simulink model "Target_Control_System"  (R2021b)
settings: Solver=FixedStepDiscrete  StartTime=0.0  StopTime=5  RelTol=1e-3
PreLoadFcn:
  | RTWConfigurationCB('preloadfcn', bdroot);
PostLoadFcn:
  | load('configuration/data_struct.mat');
  | load('configuration/fluxMaps_propMotor.mat');
  | load('configuration/parameterInit_PROP.mat');
  | load('configuration/parameterInit_PUMP.mat');
  | load('configuration/parameterInit_PITCH.mat');
  | load('configuration/parameterInit_TILT.mat');
  | %load('configuration/base_workspace_signal_definition.mat');
  | %load('resolvedatastores_to_baseworkspace_for_faster_simulation.mat');
model workspace (MAT data in the model file):
  SIMULATION_OPTIONS : Simulink.Parameter (value not decoded)
  TARGET_CODE_GEN : Simulink.Parameter (value not decoded)
  TCS_SAMPLE_FREQ_HZ : Simulink.Parameter (value not decoded)
symbols that are objects in the model workspace (value not decoded): TARGET_CODE_GEN, TCS_SAMPLE_FREQ_HZ
undefined symbols (not defined in the file): A_DQ_REF_LPF_INIT__PITCH, A_DQ_REF_LPF_INIT__PROP, A_DQ_REF_LPF_INIT__PUMP, A_DQ_REF_LPF_INIT__TILT, A_OBSERVER_CONFIDENCE_INIT__PITCH, A_OBSERVER_CONFIDENCE_INIT__PROP, A_OBSERVER_CONFIDENCE_INIT__PUMP, A_OBSERVER_CONFIDENCE_INIT__TILT, ACTUATOR_MAX_ANGLE_TRIP__PITCH, ACTUATOR_MIN_ANGLE_TRIP__PITCH, ACTUATOR_POS_SENSOR_INV_DIRECTION__PITCH, ACTUATOR_POS_SENSOR_INV_DIRECTION__TILT, ACTUATOR_POS_SENSOR_OFFSET__PITCH, ACTUATOR_POS_SENSOR_OFFSET__TILT, ADC_scaler1_baseaddr_TILT, ADC_SCALER_FLOAT_TO_FIXPOINT_EXPANSION, ANGLE_ELEC_FROM_SENSOR_OFFSET_INIT__PITCH, ANGLE_ELEC_FROM_SENSOR_OFFSET_INIT__PROP, ANGLE_ELEC_FROM_SENSOR_OFFSET_INIT__PUMP, ANGLE_ELEC_FROM_SENSOR_OFFSET_INIT__TILT, AUTO_CLEAR_FAULTS_ENABLED__PITCH, AUTO_CLEAR_FAULTS_ENABLED__PROP, AUTO_CLEAR_FAULTS_ENABLED__PUMP, AUTO_CLEAR_FAULTS_ENABLED__TILT, AUTO_CLEAR_FAULTS_WAIT_TICKS__PITCH, AUTO_CLEAR_FAULTS_WAIT_TICKS__PROP, AUTO_CLEAR_FAULTS_WAIT_TICKS__PUMP, AUTO_CLEAR_FAULTS_WAIT_TICKS__TILT, AUTO_I_ZERO_IDLE_TICKS__PITCH, AUTO_I_ZERO_IDLE_TICKS__PROP, AUTO_I_ZERO_IDLE_TICKS__PUMP, AUTO_I_ZERO_IDLE_TICKS__TILT, AUTO_I_ZERO_OFFSET_IDC_THRESHOLD__PITCH, AUTO_I_ZERO_OFFSET_IDC_THRESHOLD__PROP, AUTO_I_ZERO_OFFSET_IDC_THRESHOLD__PUMP, AUTO_I_ZERO_OFFSET_IDC_THRESHOLD__TILT, AUTO_I_ZERO_OFFSET_IPH_THRESHOLD__PITCH, AUTO_I_ZERO_OFFSET_IPH_THRESHOLD__PROP, AUTO_I_ZERO_OFFSET_IPH_THRESHOLD__PUMP, AUTO_I_ZERO_OFFSET_IPH_THRESHOLD__TILT, AUTO_SENSORLESS_SWITCHOVER_DISABLE_OMEGA, AUTO_SENSORLESS_SWITCHOVER_ENABLE_OMEGA, AUTO_SENSORLESS_SWITCHOVER_MIN_CONFIDENCE, AUXILIARY_PROTECTION_UNIT_BASEADDR__TILT, blanking_max_error_omega_INIT_PITCH, blanking_max_error_omega_INIT_TILT, blanking_max_error_position_INIT_PITCH, blanking_max_error_position_INIT_TILT, BRUTE_START_I_Q_REF_RAMP_SPEED__PITCH, BRUTE_START_I_Q_REF_RAMP_SPEED__PROP, BRUTE_START_I_Q_REF_RAMP_SPEED__PUMP, BRUTE_START_I_Q_REF_RAMP_SPEED__TILT, CONTROL_LOOP_DT_INIT__PITCH, CONTROL_LOOP_DT_INIT__PROP, CONTROL_LOOP_DT_INIT__PUMP, CONTROL_LOOP_DT_INIT__TILT, CORRECTION_FILTER_SCALE__PITCH, CORRECTION_FILTER_SCALE__PROP, CORRECTION_FILTER_SCALE__PUMP, CORRECTION_FILTER_SCALE__TILT ... (+458)
libraries: simulink x178, Reusables_Lib x24
(part 37 of 47)

== system Target_Control_System/Target_Control_System/MainLoop/pitchMotor_mainLoop/mainTask_pitch/motorTaskMainFastStep()/Control Loops - Pitch/Speed Controller Pitch/Enabled Subsystem1 ==
  oRampDataOmegaERef_.fRampOut : Inport
  Enable : EnablePort
  Constant2 : Constant  OutDataTypeStr=single  SampleTime=-1
  Data Store Read1 : DataStoreRead  DataStoreName=oPitch  DataStoreElements=oPitch.oMot_.oParam_.oPiDataRpm_.oParameter_.fKp_  IndexOptions=Index vector (dialog)  Indices=1  OutputSizes=1
  Data Store Read11 : DataStoreRead  DataStoreName=oPitch  DataStoreElements=oPitch.oMot_.oParam_.oPiDataRpm_.oParameter_.fIntMax_  IndexOptions=Index vector (dialog)  Indices=1  OutputSizes=1
  Data Store Read13 : DataStoreRead  DataStoreName=oPitch  DataStoreElements=oPitch.oMot_.oParam_.oPiDataRpm_.oParameter_.fOutMin_  IndexOptions=Index vector (dialog)  Indices=1  OutputSizes=1
  Data Store Read2 : DataStoreRead  DataStoreName=oPitch  DataStoreElements=oPitch.oMot_.oParam_.oPiDataRpm_.oParameter_.fKi_  IndexOptions=Index vector (dialog)  Indices=1  OutputSizes=1
  Data Store Read25 : DataStoreRead  DataStoreName=oPitch  DataStoreElements=oPitch.oMot_.oParam_.oPiDataRpm_.oParameter_.fOutMax_  IndexOptions=Index vector (dialog)  Indices=1  OutputSizes=1
  Data Store Read26 : DataStoreRead  DataStoreName=oPitch  DataStoreElements=oPitch.oMot_.oParam_.oPiDataRpm_.fState_  IndexOptions=Index vector (dialog)  Indices=1  OutputSizes=1
  Data Store Read27 : DataStoreRead  DataStoreName=oPitch  DataStoreElements=oPitch.oMot_.oIn_.fOmegaEObserverLpf2_  IndexOptions=Index vector (dialog)  Indices=1  OutputSizes=1
  Data Store Read5 : DataStoreRead  DataStoreName=oPitch  DataStoreElements=oPitch.oMot_.oParam_.oPiDataRpm_.oParameter_.fLoopDt_  IndexOptions=Index vector (dialog)  Indices=1  OutputSizes=1
  Data Store Read6 : DataStoreRead  DataStoreName=oPitch  DataStoreElements=oPitch.oMot_.oParam_.oPiDataRpm_.oParameter_.fIntMin_  IndexOptions=Index vector (dialog)  Indices=1  OutputSizes=1
  Data Store Write4 : DataStoreWrite  DataStoreName=oPitch  DataStoreElements=oPitch.oMot_.oState_.fIqRefFromSpeedController_  IndexOptions=Index vector (dialog)  Indices=1  OutputSizes=1
  Data Store Write6 : DataStoreWrite  DataStoreName=oPitch  DataStoreElements=oPitch.oMot_.oParam_.oPiDataRpm_.fState_  IndexOptions=Index vector (dialog)  Indices=1  OutputSizes=1
  PI Iq Current Controller : Subsystem
  fIqRefFromSpeedController : Outport
  wires:
  PI Iq Current Controller/1(fOutput) -> Data Store Write4/1, fIqRefFromSpeedController/1
  PI Iq Current Controller/2(*fpState) -> Data Store Write6/1
  oRampDataOmegaERef_.fRampOut/1 -> PI Iq Current Controller/1(fTarget)
  Data Store Read27/1 -> PI Iq Current Controller/2(fActual)
  Constant2/1 -> PI Iq Current Controller/5(fScale)
  Data Store Read25/1 -> PI Iq Current Controller/8(fOutMax)
  Data Store Read13/1 -> PI Iq Current Controller/10(fOutMin)
  Data Store Read11/1 -> PI Iq Current Controller/7(fIntMax)
  Data Store Read6/1 -> PI Iq Current Controller/9(fIntMin)
  Data Store Read5/1 -> PI Iq Current Controller/6(fLoopDt)
  Data Store Read2/1 -> PI Iq Current Controller/4(fKi)
  Data Store Read1/1 -> PI Iq Current Controller/3(fKp)

== system Target_Control_System/Target_Control_System/MainLoop/pitchMotor_mainLoop/mainTask_pitch/motorTaskMainFastStep()/Control Loops - Pitch/Speed Controller Pitch/Set Iq Ref Pitch ==
  note: // Run a low pass filter on the reference output from the speed controller.
      | // Main motivation: this is for the other inverter in dual motor servo loops, where the other inverter runs in torque
      | // mirror mode. The comms bandwidth to the other inverter is slower than the control loop. Without filter, aliasing will
      | // happen. (Example: on a quick motor deceleration there might be a brief high torque spike. If exactly this spike gets
      | // communicated across, the other inverter will apply this torque for much longer, essentially causing the inverters to
      | // fight for a few cycles.)
  fIqRefFromSpeedController : Inport
  Enable : EnablePort
  Data Store Read : DataStoreRead  DataStoreName=oPitch  DataStoreElements=oPitch.oMot_.oState_.oFilterDataForSpeedControlIqRef_.afConstantsA_.h0  IndexOptions=Index vector (dialog)  Indices=1  OutputSizes=1
  Data Store Read1 : DataStoreRead  DataStoreName=oPitch  DataStoreElements=oPitch.oMot_.oState_.oFilterDataForSpeedControlIqRef_.afConstantsA_.h1  IndexOptions=Index vector (dialog)  Indices=1  OutputSizes=1
  Data Store Read2 : DataStoreRead  DataStoreName=oPitch  DataStoreElements=oPitch.oMot_.oState_.oFilterDataForSpeedControlIqRef_.afConstantsA_.h2  IndexOptions=Index vector (dialog)  Indices=1  OutputSizes=1
  Data Store Read3 : DataStoreRead  DataStoreName=oPitch  DataStoreElements=oPitch.oMot_.oState_.oFilterDataForSpeedControlIqRef_.afConstantsB_.h0  IndexOptions=Index vector (dialog)  Indices=1  OutputSizes=1
  Data Store Read4 : DataStoreRead  DataStoreName=oPitch  DataStoreElements=oPitch.oMot_.oState_.oFilterDataForSpeedControlIqRef_.afConstantsB_.h1  IndexOptions=Index vector (dialog)  Indices=1  OutputSizes=1
  Data Store Read5 : DataStoreRead  DataStoreName=oPitch  DataStoreElements=oPitch.oMot_.oState_.oFilterDataForSpeedControlIqRef_.afConstantsB_.h2  IndexOptions=Index vector (dialog)  Indices=1  OutputSizes=1
  Data Store Read6 : DataStoreRead  DataStoreName=oPitch  DataStoreElements=oPitch.oMot_.oState_.oFilterDataForSpeedControlIqRef_.afPreviousInputs_.h0  IndexOptions=Index vector (dialog)  Indices=1  OutputSizes=1
  Data Store Read7 : DataStoreRead  DataStoreName=oPitch  DataStoreElements=oPitch.oMot_.oState_.oFilterDataForSpeedControlIqRef_.afPreviousInputs_.h1  IndexOptions=Index vector (dialog)  Indices=1  OutputSizes=1
  Data Store Read8 : DataStoreRead  DataStoreName=oPitch  DataStoreElements=oPitch.oMot_.oState_.oFilterDataForSpeedControlIqRef_.afPreviousOutputs_.h0  IndexOptions=Index vector (dialog)  Indices=1  OutputSizes=1
  Data Store Read9 : DataStoreRead  DataStoreName=oPitch  DataStoreElements=oPitch.oMot_.oState_.oFilterDataForSpeedControlIqRef_.afPreviousOutputs_.h1  IndexOptions=Index vector (dialog)  Indices=1  OutputSizes=1
  Data Store Write1 : DataStoreWrite  DataStoreName=oPitch  DataStoreElements=oPitch.oMot_.oState_.oFilterDataForSpeedControlIqRef_.fFilterOutput_  IndexOptions=Index vector (dialog)  Indices=1  OutputSizes=1
  Data Store Write2 : DataStoreWrite  DataStoreName=oPitch  DataStoreElements=oPitch.oMot_.oState_.oFilterDataForSpeedControlIqRef_.afPreviousOutputs_.h0  IndexOptions=Index vector (dialog)  Indices=1  OutputSizes=1
  Data Store Write3 : DataStoreWrite  DataStoreName=oPitch  DataStoreElements=oPitch.oMot_.oState_.oFilterDataForSpeedControlIqRef_.afPreviousOutputs_.h1  IndexOptions=Index vector (dialog)  Indices=1  OutputSizes=1
  Data Store Write4 : DataStoreWrite  DataStoreName=oPitch  DataStoreElements=oPitch.oMot_.oState_.oFilterDataForSpeedControlIqRef_.afPreviousInputs_.h0  IndexOptions=Index vector (dialog)  Indices=1  OutputSizes=1
  Data Store Write5 : DataStoreWrite  DataStoreName=oPitch  DataStoreElements=oPitch.oMot_.oState_.oFilterDataForSpeedControlIqRef_.afPreviousInputs_.h1  IndexOptions=Index vector (dialog)  Indices=1  OutputSizes=1
  Data Store Write6 : DataStoreWrite  DataStoreName=oPitch  DataStoreElements=oPitch.oMot_.oState_.fIqRefBeforeRamp_  IndexOptions=Index vector (dialog)  Indices=1  OutputSizes=1
  softwareIirFilterStep() : Subsystem
  wires:
  fIqRefFromSpeedController/1 -> softwareIirFilterStep()/1(newInput), Data Store Write6/1
  softwareIirFilterStep()/1(*afPreviousInputs1) -> Data Store Write5/1
  softwareIirFilterStep()/2(*afPreviousInputs0) -> Data Store Write4/1
  softwareIirFilterStep()/3(*afPreviousOutputs1) -> Data Store Write3/1
  softwareIirFilterStep()/4(*afPreviousOutputs0) -> Data Store Write2/1
  softwareIirFilterStep()/5(fFilterOutput) -> Data Store Write1/1
  Data Store Read6/1 -> softwareIirFilterStep()/8(afPreviousInputs0)
  Data Store Read7/1 -> softwareIirFilterStep()/9(afPreviousInputs1)
  Data Store Read8/1 -> softwareIirFilterStep()/10(afPreviousOutputs0)
  Data Store Read9/1 -> softwareIirFilterStep()/11(afPreviousOutputs1)
  Data Store Read2/1 -> softwareIirFilterStep()/7(afConstantsA2)
  Data Store Read1/1 -> softwareIirFilterStep()/6(afConstantsA1)
  Data Store Read/1 -> softwareIirFilterStep()/5(afConstantsA0)
  Data Store Read3/1 -> softwareIirFilterStep()/2(afConstantsB0)
  Data Store Read4/1 -> softwareIirFilterStep()/3(afConstantsB1)
  Data Store Read5/1 -> softwareIirFilterStep()/4(afConstantsB2)

== system Target_Control_System/Target_Control_System/MainLoop/pitchMotor_mainLoop/mainTask_pitch/motorTaskMainFastStep()/Mechanical System - Pitch/processSensors(&oPitch)/Auxiliary sensor ==
  note: // Only process this if the sensor is actually there (mostly to save time for the QI).
  Enable : EnablePort
  Add2 : Sum
  Add4 : Sum
  Constant16 : Constant  Value=pi  OutDataTypeStr=single  SampleTime=-1
  Constant17 : Constant  Value=2*pi  OutDataTypeStr=single  SampleTime=-1
  Constant3 : Constant  Value=pi  OutDataTypeStr=single  SampleTime=-1
  Constant6 : Constant  Value=2*pi  OutDataTypeStr=single  SampleTime=-1
  Data Store Read67 : DataStoreRead  DataStoreName=oPitch  DataStoreElements=oPitch.oMot_.oState_.oPosSensor_.iAuxiliarySensorInverseDirection_  IndexOptions=Index vector (dialog)  Indices=1  OutputSizes=1
  Data Store Read68 : DataStoreRead  DataStoreName=oPitch  DataStoreElements=oPitch.oMot_.oIn_.oAdcData_.fAuxiliaryEncoderFloat_  IndexOptions=Index vector (dialog)  Indices=1  OutputSizes=1
  Data Store Read91 : DataStoreRead  DataStoreName=oPitch  DataStoreElements=oPitch.oMot_.oState_.oPosSensor_.fAuxiliarySensorOffsetAngle_  IndexOptions=Index vector (dialog)  Indices=1  OutputSizes=1
  Data Store Write37 : DataStoreWrite  DataStoreName=oPitch  DataStoreElements=oPitch.oMot_.oState_.oPosSensor_.fAuxiliaryAngleFromSensor_  IndexOptions=Index vector (dialog)  Indices=1  OutputSizes=1
  Subtract3 : Sum  Inputs=+-
  Subtract4 : Sum  Inputs=+-
  Subtract5 : Sum  Inputs=-+
  Switch10 : Switch  Threshold=-pi/2.0
  Switch8 : Switch  Criteria=u2 > Threshold
  Switch9 : Switch  Criteria=u2 > Threshold  Threshold=1.5*pi
  wires:
  Switch9/1 -> Data Store Write37/1
  Data Store Read91/1 -> Add2/1
  Constant16/1 -> Subtract4/2
  Add4/1 -> Switch10/3
  Add2/1 -> Subtract5/2, Add4/1, Switch10/2, Switch10/1, Switch9/2
  Data Store Read68/1 -> Subtract3/2, Subtract4/1
  Subtract4/1 -> Switch8/3
  Data Store Read67/1 -> Switch8/2
  Subtract5/1 -> Switch9/1
  Constant6/1 -> Add4/2
  Switch10/1 -> Switch9/3
  Subtract3/1 -> Switch8/1
  Constant17/1 -> Subtract5/1
  Switch8/1 -> Add2/2
  Constant3/1 -> Subtract3/1

== system Target_Control_System/Target_Control_System/MainLoop/pitchMotor_mainLoop/mainTask_pitch/motorTaskMainFastStep()/Mechanical System - Pitch/processSensors(&oPitch)/Input (motor) side sensor ==
  note: // Ensure the angle is within -pi/2 to pi*1.5 (no loop needed, assuming 'fActuatorSensorOffsetAngle_' is within -pi to pi)
      |    // The reason for this 'skewed' wrap around angle: the tilt sensor on the linkage style tilts moves between 0 and 200 deg,
      |    // so it'd be mighty convenient if it doesn't wrap around at 180 deg. The flaps have a similar situation.
      |    // For pivot style tilt and VP, the sensor moves between -15 deg and 100 deg at most, so the the shifted wrapping point is a non-issue.
  note: // In the tilt motor on nacelles 1 and 4-6, the sensor read head is mounted to the gearbox output shaft.
      | // For every full motor rotation, the read head moves by 1/160*360 degrees = 2.25 degrees w.r.t the stator.
      | // (So with our 20 pole pairs, that is 45 degrees electrical.)
      | // We have to adjust the offset for this.
  note: //Note to future self: there is a slim chance that 'opStates->oPosSensor_.oGbx_.fCurrentOutputAngle_'
      | may need to be multiplied by -1.0F for certain hardware assemblies. Just keep it in mind.
  " " : Subsystem
  Add5 : Sum
  Add6 : Sum
  Compute Speed From Sensor : Subsystem
  Constant15 : Constant  Value=pi  OutDataTypeStr=single  SampleTime=-1
  Constant18 : Constant  Value=pi  OutDataTypeStr=single  SampleTime=-1
  Data Store Read101 : DataStoreRead  DataStoreName=oPitch  DataStoreElements=oPitch.oMot_.oState_.oPosSensor_.iMotorSensorInverseDirection_  IndexOptions=Index vector (dialog)  Indices=1  OutputSizes=1
  Data Store Read102 : DataStoreRead  DataStoreName=oPitch  DataStoreElements=oPitch.oMot_.oIn_.oAdcData_.fMotorEncoderFloat_  IndexOptions=Index vector (dialog)  Indices=1  OutputSizes=1
  Data Store Read70 : DataStoreRead  DataStoreName=oPitch  DataStoreElements=oPitch.oMot_.oState_.oPosSensor_.fAngleElecFromSensorOffset_  IndexOptions=Index vector (dialog)  Indices=1  OutputSizes=1
  Data Store Read72 : DataStoreRead  DataStoreName=oPitch  DataStoreElements=oPitch.oMot_.oParam_.fOneOverSensorPolepairs_  IndexOptions=Index vector (dialog)  Indices=1  OutputSizes=1
  Data Store Read85 : DataStoreRead  DataStoreName=oPitch  DataStoreElements=oPitch.oMot_.oState_.oPosSensor_.iAngleElecFromSensorNumOfIdenticalValues_  IndexOptions=Index vector (dialog)  Indices=1  OutputSizes=1
  Data Store Read96 : DataStoreRead  DataStoreName=oPitch  DataStoreElements=oPitch.oMot_.oState_.oPosSensor_.iTiltReadheadCompensationEnabled_  IndexOptions=Index vector (dialog)  Indices=1  OutputSizes=1
  Data Store Read98 : DataStoreRead  DataStoreName=oPitch  DataStoreElements=oPitch.oMot_.oParam_.fPolePairs_  IndexOptions=Index vector (dialog)  Indices=1  OutputSizes=1
  Data Store Write1 : DataStoreWrite  DataStoreName=oPitch  DataStoreElements=oPitch.oMot_.oState_.oPosSensor_.fAngleElecFromSensor_  IndexOptions=Index vector (dialog)  Indices=1  OutputSizes=1
  Data Store Write38 : DataStoreWrite  DataStoreName=oPitch  DataStoreElements=oPitch.oMot_.oState_.oPosSensor_.fAngleMechMotorFromSensor_  IndexOptions=Index vector (dialog)  Indices=1  OutputSizes=1
  Data Store Write40 : DataStoreWrite  DataStoreName=oPitch  DataStoreElements=oPitch.oMot_.oState_.oPosSensor_.fOmegaEFromSensor_  IndexOptions=Index vector (dialog)  Indices=1  OutputSizes=1
  Data Store Write41 : DataStoreWrite  DataStoreName=oPitch  DataStoreElements=oPitch.oMot_.oState_.oPosSensor_.fAngleElecFromSensorPrevious_  IndexOptions=Index vector (dialog)  Indices=1  OutputSizes=1
  Data Store Write42 : DataStoreWrite  DataStoreName=oPitch  DataStoreElements=oPitch.oMot_.oState_.oPosSensor_.iAngleMechToElecWrappings_  IndexOptions=Index vector (dialog)  Indices=1  OutputSizes=1
  Product : Product  Inputs=3
  Stuck Sensor Detection : Subsystem
  Subtract6 : Sum  Inputs=+-
  Subtract7 : Sum  Inputs=+-
  Switch14 : Switch  Criteria=u2 > Threshold
  Switch16 : Switch  Criteria=u2 > Threshold
  Unit Delay : UnitDelay  SampleTime=-1  HasFrameUpgradeWarning=on
  updateGbxOutput : Subsystem
  wires:
  Switch16/1 -> Product/1
  Data Store Read96/1 -> Switch16/2
  Data Store Read70/1 -> Add6/2
  Data Store Read101/1 -> Switch14/2
  Add6/1 -> " "/1(input_angle)  "angle_elec_unwrapped"
  Add5/1 -> Switch16/1
  Switch14/1 -> Data Store Write38/1, updateGbxOutput/1(fNewInputAngle), Switch16/3, Add5/2  "fAngleMechMotorFromSensor"
  " "/2(wrapped_angle) -> Unit Delay/1, Compute Speed From Sensor/2(fAngleElecFromSensor), Stuck Sensor Detection/1(fAngleElecFromSensor), Data Store Write1/1  "fAngleElecFromSensor"
  " "/1(rev_count) -> Data Store Write42/1
  Data Store Read102/1 -> Subtract7/1, Subtract6/2  "fMotorEncoderFloat"
  Data Store Read72/1 -> Product/3
  Product/1 -> Add6/1
  Data Store Read85/1 -> Stuck Sensor Detection/2(NumOfIdenticalValues)
  Compute Speed From Sensor/1(fOmegaEFromSensor) -> Data Store Write40/1
  Constant15/1 -> Subtract7/2
  Subtract6/1 -> Switch14/1
  Data Store Read98/1 -> Product/2
  Unit Delay/1 -> Stuck Sensor Detection/3(fAngleElecFromSensorPrevious), Compute Speed From Sensor/1(fAngleElecFromSensorPrevious)
  Compute Speed From Sensor/2(AngleCurrent) -> Data Store Write41/1
  Constant18/1 -> Subtract6/1
  updateGbxOutput/1(fCurrentOutputAngle) -> Add5/1
  Subtract7/1 -> Switch14/3

== system Target_Control_System/Target_Control_System/MainLoop/pitchMotor_mainLoop/mainTask_pitch/motorTaskMainFastStep()/Mechanical System - Pitch/processSensors(&oPitch)/Output (actuator) side sensor ==
  note: // Ensure the angle is within -pi/2 to pi*1.5 (no loop needed, assuming 'fActuatorSensorOffsetAngle_' is within -pi to pi)
      |    // The reason for this 'skewed' wrap around angle: the tilt sensor on the linkage style tilts moves between 0 and 200 deg,
      |    // so it'd be mighty convenient if it doesn't wrap around at 180 deg. The flaps have a similar situation.
      |    // For pivot style tilt and VP, the sensor moves between -15 deg and 100 deg at most, so the the shifted wrapping point is a non-issue.
  Add : Sum
  Add4 : Sum
  Constant16 : Constant  Value=pi  OutDataTypeStr=single  SampleTime=-1
  Constant17 : Constant  Value=2*pi  OutDataTypeStr=single  SampleTime=-1
  Constant3 : Constant  Value=pi  OutDataTypeStr=single  SampleTime=-1
  Constant6 : Constant  Value=2*pi  OutDataTypeStr=single  SampleTime=-1
  Data Store Read67 : DataStoreRead  DataStoreName=oPitch  DataStoreElements=oPitch.oMot_.oState_.oPosSensor_.iActuatorSensorInverseDirection_  IndexOptions=Index vector (dialog)  Indices=1  OutputSizes=1
  Data Store Read68 : DataStoreRead  DataStoreName=oPitch  DataStoreElements=oPitch.oMot_.oIn_.oAdcData_.fOutputEncoderFloat_  IndexOptions=Index vector (dialog)  Indices=1  OutputSizes=1
  Data Store Read91 : DataStoreRead  DataStoreName=oPitch  DataStoreElements=oPitch.oMot_.oState_.oPosSensor_.fActuatorSensorOffsetAngle_  IndexOptions=Index vector (dialog)  Indices=1  OutputSizes=1
  Data Store Write37 : DataStoreWrite  DataStoreName=oPitch  DataStoreElements=oPitch.oMot_.oState_.oPosSensor_.fActuatorAngleFromSensor_  IndexOptions=Index vector (dialog)  Indices=1  OutputSizes=1
  Subtract : Sum  Inputs=+-
  Subtract1 : Sum  Inputs=+-
  Subtract2 : Sum  Inputs=-+
  Switch10 : Switch  Threshold=-pi/2.0
  Switch8 : Switch  Criteria=u2 > Threshold
  Switch9 : Switch  Criteria=u2 > Threshold  Threshold=1.5*pi
  wires:
  Constant6/1 -> Add4/2
  Constant17/1 -> Subtract2/1
  Subtract2/1 -> Switch9/1
  Data Store Read91/1 -> Add/1
  Subtract/1 -> Switch8/1
  Switch10/1 -> Switch9/3
  Switch9/1 -> Data Store Write37/1
  Constant3/1 -> Subtract/1
  Constant16/1 -> Subtract1/2
  Data Store Read68/1 -> Subtract/2, Subtract1/1
  Subtract1/1 -> Switch8/3
  Data Store Read67/1 -> Switch8/2
  Switch8/1 -> Add/2
  Add/1 -> Subtract2/2, Add4/1, Switch10/2, Switch10/1, Switch9/2
  Add4/1 -> Switch10/3

== system Target_Control_System/Target_Control_System/MainLoop/pitchMotor_mainLoop/mainTask_pitch/motorTaskMainFastStep()/Motor Acceleration - Pitch/First filter stage/softwareIirFilterStep() ==
  newInput : Inport
  afConstantsB0 : Inport  Port=2
  afConstantsB1 : Inport  Port=3
  afConstantsB2 : Inport  Port=4
  afConstantsA0 : Inport  Port=5
  afConstantsA1 : Inport  Port=6
  afConstantsA2 : Inport  Port=7
  afPreviousInputs0 : Inport  Port=8
  afPreviousInputs1 : Inport  Port=9
  afPreviousOutputs0 : Inport  Port=10
  afPreviousOutputs1 : Inport  Port=11
  Add : Sum  Inputs=+++--
  Constant : Constant  Value=0  OutDataTypeStr=single  SampleTime=-1
  Constant1 : Constant  Value=0  OutDataTypeStr=single  SampleTime=-1
  Divide{,1..5} (6 alike) : Product  Inputs=**
  IsInf : RelationalOperator  Operator=isInf  OutDataTypeStr=boolean  RndMeth=Simplest
  IsInf1 : RelationalOperator  Operator=isInf  OutDataTypeStr=boolean  RndMeth=Simplest
  IsNaN : RelationalOperator  Operator=isNaN  OutDataTypeStr=boolean  RndMeth=Simplest
  IsNaN1 : RelationalOperator  Operator=isNaN  OutDataTypeStr=boolean  RndMeth=Simplest
  Switch{,1..3} (4 alike) : Switch  Criteria=u2 > Threshold
  *afPreviousInputs1 : Outport
  *afPreviousInputs0 : Outport  Port=2
  *afPreviousOutputs1 : Outport  Port=3
  *afPreviousOutputs0 : Outport  Port=4
  fFilterOutput : Outport  Port=5
  wires:
  Switch3/1 -> Divide5/1, *afPreviousOutputs0/1
  IsInf1/1 -> Switch3/2
  IsNaN1/1 -> Switch2/2
  Constant1/1 -> Switch2/1, Switch3/1
  Switch2/1 -> IsInf1/1, Switch3/3
  Add/1 -> IsNaN1/1, Switch2/3  "fOutput"
  Switch1/1 -> Divide/1, *afPreviousInputs0/1
  Switch/1 -> IsInf/1, Switch1/3
  IsInf/1 -> Switch1/2
  Constant/1 -> Switch/1, Switch1/1
  IsNaN/1 -> Switch/2
  Divide5/1 -> fFilterOutput/1
  afConstantsA0/1 -> Divide5/2
  afPreviousOutputs1/1 -> Divide4/1
  afConstantsA2/1 -> Divide4/2
  afPreviousOutputs0/1 -> Divide3/1, *afPreviousOutputs1/1
  afConstantsA1/1 -> Divide3/2
  afPreviousInputs1/1 -> Divide2/1
  afConstantsB2/1 -> Divide2/2
  Divide4/1 -> Add/5
  Divide3/1 -> Add/4
  Divide/1 -> Add/1
  Divide1/1 -> Add/2
  Divide2/1 -> Add/3
  afPreviousInputs0/1 -> Divide1/1, *afPreviousInputs1/1
  afConstantsB1/1 -> Divide1/2
  newInput/1 -> IsNaN/1, Switch/3
  afConstantsB0/1 -> Divide/2

== system Target_Control_System/Target_Control_System/MainLoop/pitchMotor_mainLoop/mainTask_pitch/motorTaskMainFastStep()/Observer Confidence - Pitch/Automatic switching to sensorless/Switch to sensored?  ==
  fObserverConfidence : Inport
  Action Port : ActionPort
  Abs1 : Abs
  Data Store Read28 : DataStoreRead  DataStoreName=oPitch  DataStoreElements=oPitch.oMot_.oIn_.fOmegaEObserverRaw2_  IndexOptions=Index vector (dialog)  Indices=1  OutputSizes=1
  Data Store Read29 : DataStoreRead  DataStoreName=oPitch  DataStoreElements=oPitch.oMot_.oParam_.fAutoSensorlessSwitchoverDisableOmega_  IndexOptions=Index vector (dialog)  Indices=1  OutputSizes=1
  Data Store Read42 : DataStoreRead  DataStoreName=oPitch  DataStoreElements=oPitch.oMot_.oParam_.fAutoSensorlessSwitchoverMinConfidence_  IndexOptions=Index vector (dialog)  Indices=1  OutputSizes=1
  Less Than : RelationalOperator  Operator=<  OutDataTypeStr=boolean  RndMeth=Simplest
  Less Than1 : RelationalOperator  Operator=<  OutDataTypeStr=boolean  RndMeth=Simplest
  OR : Logic  Operator=OR  AllPortsSameDT=off  OutDataTypeStr=boolean
  Switch to sensored : Subsystem  TreatAsAtomicUnit=on
  wires:
  OR/1 -> Switch to sensored/Enable
  fObserverConfidence/1 -> Less Than1/1
  Data Store Read29/1 -> Less Than/2
  Data Store Read42/1 -> Less Than1/2
  Abs1/1 -> Less Than/1
  Less Than/1 -> OR/1
  Data Store Read28/1 -> Abs1/1
  Less Than1/1 -> OR/2

== system Target_Control_System/Target_Control_System/MainLoop/pitchMotor_mainLoop/mainTask_pitch/motorTaskMainFastStep()/Observer Confidence - Pitch/Automatic switching to sensorless/Switch to sensorless? ==
  fObserverConfidence : Inport
  Action Port : ActionPort
  Abs1 : Abs
  Data Store Read28 : DataStoreRead  DataStoreName=oPitch  DataStoreElements=oPitch.oMot_.oIn_.fOmegaEObserverRaw2_  IndexOptions=Index vector (dialog)  Indices=1  OutputSizes=1
  Data Store Read29 : DataStoreRead  DataStoreName=oPitch  DataStoreElements=oPitch.oMot_.oParam_.fAutoSensorlessSwitchoverEnableOmega_  IndexOptions=Index vector (dialog)  Indices=1  OutputSizes=1
  Data Store Read42 : DataStoreRead  DataStoreName=oPitch  DataStoreElements=oPitch.oMot_.oParam_.fAutoSensorlessSwitchoverMinConfidence_  IndexOptions=Index vector (dialog)  Indices=1  OutputSizes=1
  Less Than : RelationalOperator  Operator=>  OutDataTypeStr=boolean  RndMeth=Simplest
  Less Than1 : RelationalOperator  Operator=>  OutDataTypeStr=boolean  RndMeth=Simplest
  OR : Logic  AllPortsSameDT=off  OutDataTypeStr=boolean
  Switch to sensorless : Subsystem  TreatAsAtomicUnit=on
  wires:
  Less Than/1 -> OR/1
  Data Store Read42/1 -> Less Than1/2
  Less Than1/1 -> OR/2
  fObserverConfidence/1 -> Less Than1/1
  Data Store Read29/1 -> Less Than/2
  Data Store Read28/1 -> Abs1/1
  Abs1/1 -> Less Than/1
  OR/1 -> Switch to sensorless/Enable

== system Target_Control_System/Target_Control_System/MainLoop/pitchMotor_mainLoop/mainTask_pitch/motorTaskMainFastStep()/Software Overcurrent Protection - Pitch/checkForHwOvercurrents(&oPitch)/gateDriverStatus ==
  note: 1) Add Subsystem or Model blocks as valid variant choices.
      | 2) You cannot connect blocks at this level. At simulation, connectivity is automatically
      | determined, based on the active variant and port name matching.
  DoNotIncludeCustomCode : Subsystem  TreatAsAtomicUnit=on  VariantControl=TARGET_CODE_GEN == 0
  IncludeCustomCode : Subsystem  TreatAsAtomicUnit=on  VariantControl=(default)

== system Target_Control_System/Target_Control_System/MainLoop/propMotor_mainLoop/Decimation gate for 5000 Hz Prop/motorTaskProcessExternalSetpoints(&oProp)/Subsystem3/Subsystem/Subsystem ==
  Enable : EnablePort
  Data Store Read1 : DataStoreRead  DataStoreName=oProp  DataStoreElements=oProp.oMot_.oParam_.fIqSetpointMax_  IndexOptions=Index vector (dialog)  Indices=1  OutputSizes=1
  Data Store Read68 : DataStoreRead  DataStoreName=oProp  DataStoreElements=oProp.oMot_.oIn_.fIqSetpoint_  IndexOptions=Index vector (dialog)  Indices=1  OutputSizes=1
  Data Store Read74 : DataStoreRead  DataStoreName=oProp  DataStoreElements=oProp.oMot_.oParam_.fIqSetpointMax_  IndexOptions=Index vector (dialog)  Indices=1  OutputSizes=1
  Data Store Read81 : DataStoreRead  DataStoreName=oProp  DataStoreElements=oProp.oMot_.oParam_.fDynILimIntegratorLeakageFactor_  IndexOptions=Index vector (dialog)  Indices=1  OutputSizes=1
  Data Store Write19 : DataStoreWrite  DataStoreName=oProp  DataStoreElements=oProp.oMot_.oState_.fIqRefBeforeRamp_  IndexOptions=Index vector (dialog)  Indices=1  OutputSizes=1
  Dynamic Current Limiting Prop : Subsystem  TreatAsAtomicUnit=on
  Gain2 : Gain  Gain=-1
  Saturation Dynamic : simulink/Discontinuities/Saturation Dynamic  OutMin=[]  OutMax=[]  OutDataTypeStr=Inherit: Same as second input  OutDataType=fixdt(1, 16)  OutScaling=2^-10  DoSatur=off
  Switch4 : Switch  Criteria=u2 > Threshold
  wires:
  Dynamic Current Limiting Prop/1(fIqRefBeforeRamp_) -> Switch4/1
  Switch4/1 -> Data Store Write19/1
  Data Store Read81/1 -> Dynamic Current Limiting Prop/Enable, Switch4/2
  Gain2/1 -> Saturation Dynamic/3
  Data Store Read74/1 -> Saturation Dynamic/1
  Data Store Read68/1 -> Saturation Dynamic/2
  Data Store Read1/1 -> Gain2/1
  Saturation Dynamic/1 -> Switch4/3

== system Target_Control_System/Target_Control_System/MainLoop/propMotor_mainLoop/Decimation gate for 5000 Hz Prop/motorTaskProcessExternalSetpoints(&oProp)/Subsystem3/Subsystem1/Subsystem ==
  Input : Inport
  Enable : EnablePort
  Data Store Read1 : DataStoreRead  DataStoreName=oProp  DataStoreElements=oProp.oMot_.oParam_.fISetpointMax_  IndexOptions=Index vector (dialog)  Indices=1  OutputSizes=1
  Data Store Read2 : DataStoreRead  DataStoreName=oProp  DataStoreElements=oProp.oMot_.oParam_.fISetpointMax_  IndexOptions=Index vector (dialog)  Indices=1  OutputSizes=1
  Data Store Write1 : DataStoreWrite  DataStoreName=oProp  DataStoreElements=oProp.oMot_.oState_.fIdExternalSetpoint_  IndexOptions=Index vector (dialog)  Indices=1  OutputSizes=1
  Gain2 : Gain  Gain=-1
  Saturation Dynamic : simulink/Discontinuities/Saturation Dynamic  OutMin=[]  OutMax=[]  OutDataTypeStr=Inherit: Same as second input  OutDataType=fixdt(1, 16)  OutScaling=2^-10  DoSatur=off
  wires:
  Data Store Read1/1 -> Gain2/1
  Data Store Read2/1 -> Saturation Dynamic/1
  Gain2/1 -> Saturation Dynamic/3
  Input/1 -> Saturation Dynamic/2
  Saturation Dynamic/1 -> Data Store Write1/1

== system Target_Control_System/Target_Control_System/MainLoop/propMotor_mainLoop/Decimation gate for 5000 Hz Prop/motorTaskProcessExternalSetpoints(&oProp)/Subsystem3/Subsystem2/Subsystem ==
  Enable : EnablePort
  Data Store Read2 : DataStoreRead  DataStoreName=oProp  DataStoreElements=oProp.oMot_.oIn_.fRpmSetpoint_  IndexOptions=Index vector (dialog)  Indices=1  OutputSizes=1
  Data Store Read3 : DataStoreRead  DataStoreName=oProp  DataStoreElements=oProp.oMot_.oParam_.fOmegaESetpointMax_  IndexOptions=Index vector (dialog)  Indices=1  OutputSizes=1
  Data Store Read4 : DataStoreRead  DataStoreName=oProp  DataStoreElements=oProp.oMot_.oParam_.fPolePairs_  IndexOptions=Index vector (dialog)  Indices=1  OutputSizes=1
  Data Store Read74 : DataStoreRead  DataStoreName=oProp  DataStoreElements=oProp.oMot_.oParam_.fOmegaESetpointMax_  IndexOptions=Index vector (dialog)  Indices=1  OutputSizes=1
  Data Store Write1 : DataStoreWrite  DataStoreName=oProp  DataStoreElements=oProp.oMot_.oState_.oRampDataOmegaERef_.fSetpoint_  IndexOptions=Index vector (dialog)  Indices=1  OutputSizes=1
  Gain : Gain  Gain=-1
  Product : Product  Inputs=3
  Saturation Dynamic : simulink/Discontinuities/Saturation Dynamic  OutMin=[]  OutMax=[]  OutDataTypeStr=Inherit: Same as second input  OutDataType=fixdt(1, 16)  OutScaling=2^-10  DoSatur=off
  const1 : Constant  Value=0.10471975512  OutDataTypeStr=single  SampleTime=-1
  wires:
  Saturation Dynamic/1 -> Data Store Write1/1
  Product/1 -> Saturation Dynamic/2
  Data Store Read3/1 -> Gain/1
  Gain/1 -> Saturation Dynamic/3
  Data Store Read74/1 -> Saturation Dynamic/1
  const1/1 -> Product/2
  Data Store Read4/1 -> Product/3
  Data Store Read2/1 -> Product/1

== system Target_Control_System/Target_Control_System/MainLoop/propMotor_mainLoop/Decimation gate for 5000 Hz Prop/motorTaskProcessExternalSetpoints(&oProp)/Subsystem3/Subsystem3/Subsystem ==
  Enable : EnablePort
  Current Limiting Prop : Subsystem  TreatAsAtomicUnit=on
  Data Store Read2 : DataStoreRead  DataStoreName=oProp  DataStoreElements=oProp.oMot_.oIn_.fPosSetpoint_  IndexOptions=Index vector (dialog)  Indices=1  OutputSizes=1
  Data Store Read85 : DataStoreRead  DataStoreName=oProp  DataStoreElements=oProp.oMot_.oState_.uiDriveState_  IndexOptions=Index vector (dialog)  Indices=1  OutputSizes=1
  Data Store Write1 : DataStoreWrite  DataStoreName=oProp  DataStoreElements=oProp.oMot_.oState_.oRampDataPos_.fSetpoint_  IndexOptions=Index vector (dialog)  Indices=1  OutputSizes=1
  Equal13 : RelationalOperator  Operator=~=  OutDataTypeStr=boolean  RndMeth=Simplest
  const17 : Constant  Value=228  OutDataTypeStr=uint32  SampleTime=-1
  wires:
  Equal13/1 -> Current Limiting Prop/Enable
  const17/1 -> Equal13/1
  Data Store Read85/1 -> Equal13/2
  Data Store Read2/1 -> Data Store Write1/1, Current Limiting Prop/1(oRampDataPos_.fSetpoint_)

== system Target_Control_System/Target_Control_System/MainLoop/pumpMotor_mainLoop/Decimation gate for 5000 Hz Pump/motorTaskProcessExternalSetpoints(&oPump)/Subsystem3/Subsystem/Subsystem ==
  Enable : EnablePort
  Data Store Read1 : DataStoreRead  DataStoreName=oPump  DataStoreElements=oPump.oMot_.oParam_.fIqSetpointMax_  IndexOptions=Index vector (dialog)  Indices=1  OutputSizes=1
  Data Store Read68 : DataStoreRead  DataStoreName=oPump  DataStoreElements=oPump.oMot_.oIn_.fIqSetpoint_  IndexOptions=Index vector (dialog)  Indices=1  OutputSizes=1
  Data Store Read74 : DataStoreRead  DataStoreName=oPump  DataStoreElements=oPump.oMot_.oParam_.fIqSetpointMax_  IndexOptions=Index vector (dialog)  Indices=1  OutputSizes=1
  Data Store Read81 : DataStoreRead  DataStoreName=oPump  DataStoreElements=oPump.oMot_.oParam_.fDynILimIntegratorLeakageFactor_  IndexOptions=Index vector (dialog)  Indices=1  OutputSizes=1
  Data Store Write19 : DataStoreWrite  DataStoreName=oPump  DataStoreElements=oPump.oMot_.oState_.fIqRefBeforeRamp_  IndexOptions=Index vector (dialog)  Indices=1  OutputSizes=1
  Dynamic Current Limiting Pump : Subsystem  TreatAsAtomicUnit=on
  Gain2 : Gain  Gain=-1
  Saturation Dynamic : simulink/Discontinuities/Saturation Dynamic  OutMin=[]  OutMax=[]  OutDataTypeStr=Inherit: Same as second input  OutDataType=fixdt(1, 16)  OutScaling=2^-10  DoSatur=off
  Switch4 : Switch  Criteria=u2 > Threshold
  wires:
  Dynamic Current Limiting Pump/1(fIqRefBeforeRamp_) -> Switch4/1
  Switch4/1 -> Data Store Write19/1
  Data Store Read81/1 -> Dynamic Current Limiting Pump/Enable, Switch4/2
  Gain2/1 -> Saturation Dynamic/3
  Data Store Read74/1 -> Saturation Dynamic/1
  Data Store Read68/1 -> Saturation Dynamic/2
  Data Store Read1/1 -> Gain2/1
  Saturation Dynamic/1 -> Switch4/3

== system Target_Control_System/Target_Control_System/MainLoop/pumpMotor_mainLoop/Decimation gate for 5000 Hz Pump/motorTaskProcessExternalSetpoints(&oPump)/Subsystem3/Subsystem1/Subsystem ==
  Input : Inport
  Enable : EnablePort
  Data Store Read1 : DataStoreRead  DataStoreName=oPump  DataStoreElements=oPump.oMot_.oParam_.fIqSetpointMax_  IndexOptions=Index vector (dialog)  Indices=1  OutputSizes=1
  Data Store Read74 : DataStoreRead  DataStoreName=oPump  DataStoreElements=oPump.oMot_.oParam_.fIqSetpointMax_  IndexOptions=Index vector (dialog)  Indices=1  OutputSizes=1
  Data Store Write1 : DataStoreWrite  DataStoreName=oPump  DataStoreElements=oPump.oMot_.oState_.fIdExternalSetpoint_  IndexOptions=Index vector (dialog)  Indices=1  OutputSizes=1
  Gain2 : Gain  Gain=-1
  Saturation Dynamic : simulink/Discontinuities/Saturation Dynamic  OutMin=[]  OutMax=[]  OutDataTypeStr=Inherit: Same as second input  OutDataType=fixdt(1, 16)  OutScaling=2^-10  DoSatur=off
  wires:
  Data Store Read1/1 -> Gain2/1
  Data Store Read74/1 -> Saturation Dynamic/1
  Gain2/1 -> Saturation Dynamic/3
  Input/1 -> Saturation Dynamic/2
  Saturation Dynamic/1 -> Data Store Write1/1

== system Target_Control_System/Target_Control_System/MainLoop/pumpMotor_mainLoop/Decimation gate for 5000 Hz Pump/motorTaskProcessExternalSetpoints(&oPump)/Subsystem3/Subsystem2/Subsystem ==
  Enable : EnablePort
  Data Store Read1 : DataStoreRead  DataStoreName=oPump  DataStoreElements=oPump.oMot_.oParam_.fPolePairs_  IndexOptions=Index vector (dialog)  Indices=1  OutputSizes=1
  Data Store Read2 : DataStoreRead  DataStoreName=oPump  DataStoreElements=oPump.oMot_.oIn_.fRpmSetpoint_  IndexOptions=Index vector (dialog)  Indices=1  OutputSizes=1
  Data Store Read3 : DataStoreRead  DataStoreName=oPump  DataStoreElements=oPump.oMot_.oParam_.fOmegaESetpointMax_  IndexOptions=Index vector (dialog)  Indices=1  OutputSizes=1
  Data Store Read74 : DataStoreRead  DataStoreName=oPump  DataStoreElements=oPump.oMot_.oParam_.fOmegaESetpointMax_  IndexOptions=Index vector (dialog)  Indices=1  OutputSizes=1
  Data Store Write1 : DataStoreWrite  DataStoreName=oPump  DataStoreElements=oPump.oMot_.oState_.oRampDataOmegaERef_.fSetpoint_  IndexOptions=Index vector (dialog)  Indices=1  OutputSizes=1
  Gain : Gain  Gain=-1
  Product : Product  Inputs=3
  Saturation Dynamic : simulink/Discontinuities/Saturation Dynamic  OutMin=[]  OutMax=[]  OutDataTypeStr=Inherit: Same as second input  OutDataType=fixdt(1, 16)  OutScaling=2^-10  DoSatur=off
  const1 : Constant  Value=0.10471975512  OutDataTypeStr=single  SampleTime=-1
  wires:
  Saturation Dynamic/1 -> Data Store Write1/1
  Product/1 -> Saturation Dynamic/2
  Data Store Read3/1 -> Gain/1
  Gain/1 -> Saturation Dynamic/3
  Data Store Read74/1 -> Saturation Dynamic/1
  const1/1 -> Product/2
  Data Store Read1/1 -> Product/3
  Data Store Read2/1 -> Product/1

== system Target_Control_System/Target_Control_System/MainLoop/pumpMotor_mainLoop/Decimation gate for 5000 Hz Pump/motorTaskProcessExternalSetpoints(&oPump)/Subsystem3/Subsystem3/Subsystem ==
  Enable : EnablePort
  Data Store Read2 : DataStoreRead  DataStoreName=oPump  DataStoreElements=oPump.oMot_.oIn_.fPosSetpoint_  IndexOptions=Index vector (dialog)  Indices=1  OutputSizes=1
  Data Store Read85 : DataStoreRead  DataStoreName=oPump  DataStoreElements=oPump.oMot_.oState_.uiDriveState_  IndexOptions=Index vector (dialog)  Indices=1  OutputSizes=1
  Data Store Write1 : DataStoreWrite  DataStoreName=oPump  DataStoreElements=oPump.oMot_.oState_.oRampDataPos_.fSetpoint_  IndexOptions=Index vector (dialog)  Indices=1  OutputSizes=1
  Dynamic Current Limiting Pump : Subsystem  TreatAsAtomicUnit=on
  Equal13 : RelationalOperator  Operator=~=  OutDataTypeStr=boolean  RndMeth=Simplest
  const17 : Constant  Value=228  OutDataTypeStr=uint32  SampleTime=-1
  wires:
  Equal13/1 -> Dynamic Current Limiting Pump/Enable
  const17/1 -> Equal13/1
  Data Store Read85/1 -> Equal13/2
  Data Store Read2/1 -> Data Store Write1/1, Dynamic Current Limiting Pump/1(oRampDataPos_.fSetpoint_)

== system Target_Control_System/Target_Control_System/MainLoop/pumpMotor_mainLoop/motorTaskMainFastStep(&oPump)/Control Loops - Pump/Subsystem/Set Iq Ref Pump/softwareIirFilterStep() ==
  newInput : Inport
  afConstantsB0 : Inport  Port=2
  afConstantsB1 : Inport  Port=3
  afConstantsB2 : Inport  Port=4
  afConstantsA0 : Inport  Port=5
  afConstantsA1 : Inport  Port=6
  afConstantsA2 : Inport  Port=7
  afPreviousInputs0 : Inport  Port=8
  afPreviousInputs1 : Inport  Port=9
  afPreviousOutputs0 : Inport  Port=10
  afPreviousOutputs1 : Inport  Port=11
  Add : Sum  Inputs=+++--
  Constant : Constant  Value=0  OutDataTypeStr=single
  Constant1 : Constant  Value=0  OutDataTypeStr=single
  Divide{,1..5} (6 alike) : Product  Inputs=**
  IsInf : RelationalOperator  Operator=isInf  OutDataTypeStr=boolean  RndMeth=Simplest
  IsInf1 : RelationalOperator  Operator=isInf  OutDataTypeStr=boolean  RndMeth=Simplest
  IsNaN : RelationalOperator  Operator=isNaN  OutDataTypeStr=boolean  RndMeth=Simplest
  IsNaN1 : RelationalOperator  Operator=isNaN  OutDataTypeStr=boolean  RndMeth=Simplest
  Switch{,1..3} (4 alike) : Switch  Criteria=u2 > Threshold
  *afPreviousInputs1 : Outport
  *afPreviousInputs0 : Outport  Port=2
  *afPreviousOutputs1 : Outport  Port=3
  *afPreviousOutputs0 : Outport  Port=4
  fFilterOutput : Outport  Port=5
  wires:
  Switch3/1 -> Divide5/1, *afPreviousOutputs0/1
  IsInf1/1 -> Switch3/2
  IsNaN1/1 -> Switch2/2
  Constant1/1 -> Switch2/1, Switch3/1
  Switch2/1 -> IsInf1/1, Switch3/3
  Add/1 -> IsNaN1/1, Switch2/3  "fOutput"
  Switch1/1 -> Divide/1, *afPreviousInputs0/1
  Switch/1 -> IsInf/1, Switch1/3
  IsInf/1 -> Switch1/2
  Constant/1 -> Switch/1, Switch1/1
  IsNaN/1 -> Switch/2
  Divide5/1 -> fFilterOutput/1
  afConstantsA0/1 -> Divide5/2
  afPreviousOutputs1/1 -> Divide4/1
  afConstantsA2/1 -> Divide4/2
  afPreviousOutputs0/1 -> Divide3/1, *afPreviousOutputs1/1
  afConstantsA1/1 -> Divide3/2
  afPreviousInputs1/1 -> Divide2/1
  afConstantsB2/1 -> Divide2/2
  Divide4/1 -> Add/5
  Divide3/1 -> Add/4
  Divide/1 -> Add/1
  Divide1/1 -> Add/2
  Divide2/1 -> Add/3
  afPreviousInputs0/1 -> Divide1/1, *afPreviousInputs1/1
  afConstantsB1/1 -> Divide1/2
  newInput/1 -> IsNaN/1, Switch/3
  afConstantsB0/1 -> Divide/2

== system Target_Control_System/Target_Control_System/MainLoop/pumpMotor_mainLoop/motorTaskMainFastStep(&oPump)/Control Loops - Pump/Subsystem/piControllerStep(&oPiDataRpm_)/oPiDataRpm_ ==
  fActual : Inport
  fTarget : Inport  Port=2
  fKp : Inport  Port=3
  fKi : Inport  Port=4
  fScale : Inport  Port=5
  fLoopDt : Inport  Port=6
  fIntMax : Inport  Port=7
  fOutMax : Inport  Port=8
  fIntMin : Inport  Port=9
  fOutMin : Inport  Port=10
  fState : Inport  Port=11
  Add : Sum  Inputs=|++
  Mux : Mux  Inputs=3
  Mux1 : Mux  Inputs=3
  Product : Product
  Saturation Dynamic : simulink/Discontinuities/Saturation Dynamic  OutMin=[]  OutMax=[]  OutDataTypeStr=Inherit: Same as second input  OutDataType=fixdt(1, 16)  OutScaling=2^-10  DoSatur=off
  Saturation Dynamic1 : simulink/Discontinuities/Saturation Dynamic  OutMin=[]  OutMax=[]  OutDataTypeStr=Inherit: Same as second input  OutDataType=fixdt(1, 16)  OutScaling=2^-10  DoSatur=off
  Scope3 : Scope  NumInputPorts=6
  Sum1 : Sum  Inputs=++|
  Sum22 : Sum  Inputs=-+|
  fError * fKi_ * fScale : Fcn  Expr=u(1)*u(2)*u(3)
  fError * fKp_ * fScale1 : Fcn  Expr=u(1)*u(2)*u(3)
  fOutput : Outport
  *fpState : Outport  Port=2
  wires:
  fLoopDt/1 -> Product/2
  fOutMax/1 -> Saturation Dynamic1/1
  fOutMin/1 -> Saturation Dynamic1/3
  fIntMin/1 -> Saturation Dynamic/3
  fIntMax/1 -> Saturation Dynamic/1
  Add/1 -> Saturation Dynamic/2
  fState/1 -> Add/2
  Product/1 -> Add/1
  Mux1/1 -> fError * fKp_ * fScale1/1
  fKi/1 -> Mux/2
  fScale/1 -> Mux/1, Mux1/3
  fKp/1 -> Mux1/2
  Mux/1 -> fError * fKi_ * fScale/1
  Saturation Dynamic1/1 -> fOutput/1, Scope3/6
  Sum1/1 -> Saturation Dynamic1/2  "fError"
  fError * fKp_ * fScale1/1 -> Sum1/1, Scope3/4
  Saturation Dynamic/1 -> Scope3/5, *fpState/1, Sum1/2  "*fpState"
  fActual/1 -> Sum22/1, Scope3/2
  fTarget/1 -> Sum22/2, Scope3/1
  fError * fKi_ * fScale/1 -> Product/1
  Sum22/1 -> Scope3/3, Mux/3, Mux1/1  "fError"

== system Target_Control_System/Target_Control_System/MainLoop/pumpMotor_mainLoop/motorTaskMainFastStep(&oPump)/Control Loops - Pump/Subsystem/pid2ControllerStep(&oPid2DataRpmCtrl_)/pid2ControllerStep(oPidDataRpmCtrl) ==
  fActual : Inport
  fTarget : Inport  Port=2
  fpState : Inport  Port=3
  fActualDt : Inport  Port=4
  fKp : Inport  Port=5
  fKi : Inport  Port=6
  fKd : Inport  Port=7
  fIntMin : Inport  Port=8
  fIntMax : Inport  Port=9
  fDMin : Inport  Port=10
  fDMax : Inport  Port=11
  fOutMin : Inport  Port=12
  fOutMax : Inport  Port=13
  fLoopDt : Inport  Port=14
  ipInhibitTarget : Inport  Port=15
  fBlankingMaxError : Inport  Port=16
  fLargeErrorThresholdNegative : Inport  Port=17
  fLargeErrorThresholdPositive : Inport  Port=18
  fErrorReduction : Inport  Port=19
  fIntegratorLeakFactor : Inport  Port=20
  Abs : Abs
  Abs1 : Abs
  Add : Sum  Inputs=|++
  Constant : Constant  Value=0  OutDataTypeStr=single  SampleTime=-1
  Constant1 : Constant  Value=0  OutDataTypeStr=int32  SampleTime=-1
  Constant2 : Constant  Value=-1  OutDataTypeStr=int32  SampleTime=-1
  Constant3 : Constant  Value=0  OutDataTypeStr=single  SampleTime=-1
  Constant4 : Constant  Value=0  OutDataTypeStr=single  SampleTime=-1
  Constant5 : Constant  OutDataTypeStr=single  SampleTime=-1
  Constant6 : Constant  OutDataTypeStr=int32  SampleTime=-1
  Divide : Product  Inputs=**
  Divide1 : Product  Inputs=**
  GreaterThan : RelationalOperator  Operator=>  OutDataTypeStr=boolean  RndMeth=Simplest
  GreaterThan1 : RelationalOperator  Operator=<  OutDataTypeStr=boolean  RndMeth=Simplest
  GreaterThan2 : RelationalOperator  OutDataTypeStr=boolean  RndMeth=Simplest
  GreaterThan3 : RelationalOperator  Operator=>  OutDataTypeStr=boolean  RndMeth=Simplest
  GreaterThan4 : RelationalOperator  Operator=>  OutDataTypeStr=boolean  RndMeth=Simplest
  GreaterThan5 : RelationalOperator  Operator=<  OutDataTypeStr=boolean  RndMeth=Simplest
  GreaterThan6 : RelationalOperator  Operator=<  OutDataTypeStr=boolean  RndMeth=Simplest
  OR1 : Logic  AllPortsSameDT=off  OutDataTypeStr=boolean
  OR2 : Logic  AllPortsSameDT=off  OutDataTypeStr=boolean
  OR3 : Logic  Operator=OR  AllPortsSameDT=off  OutDataTypeStr=boolean
  Product{,1..5} (6 alike) : Product
  Saturation : Saturate  UpperLimit=inf  LowerLimit=0
  Saturation Dynamic : simulink/Discontinuities/Saturation Dynamic  OutMin=[]  OutMax=[]  OutDataTypeStr=Inherit: Same as second input  OutDataType=fixdt(1, 16)  OutScaling=2^-10  DoSatur=off
  Saturation Dynamic1 : simulink/Discontinuities/Saturation Dynamic  OutMin=[]  OutMax=[]  OutDataTypeStr=Inherit: Same as second input  OutDataType=fixdt(1, 16)  OutScaling=2^-10  DoSatur=off
  Saturation Dynamic2 : simulink/Discontinuities/Saturation Dynamic  OutMin=[]  OutMax=[]  OutDataTypeStr=Inherit: Same as second input  OutDataType=fixdt(1, 16)  OutScaling=2^-10  DoSatur=off
  Sign : Signum
  Sum : Sum  Inputs=|++
  Sum2 : Sum  Inputs=-+|
  Sum22 : Sum  Inputs=-+|
  Sum4 : Sum  Inputs=-+|
  Switch{,1..3} (4 alike) : Switch  Criteria=u2 > Threshold
  Unit Delay2 : UnitDelay  SampleTime=-1  HasFrameUpgradeWarning=on
  iLargeErrorPresent : Outport
  fITerm : Outport  Port=2
  fDTerm : Outport  Port=3
  fPTerm : Outport  Port=4
  fOutput : Outport  Port=5
  *fpState : Outport  Port=6
  wires:
  Switch/1 -> Switch3/3
  Switch3/1 -> iLargeErrorPresent/1
  Constant6/1 -> Switch3/1
  GreaterThan/1 -> Switch3/2
  Sum/1 -> Saturation Dynamic1/2
  Product5/1 -> Sum/2
  Product4/1 -> fPTerm/1, Sum/1
  fKp/1 -> Product4/1
  Saturation Dynamic2/1 -> Product5/1, fDTerm/1  "fDTerm"
  fDMax/1 -> Saturation Dynamic2/1
  fDMin/1 -> Saturation Dynamic2/3
  Product3/1 -> Saturation Dynamic2/2  "fDTerm"
  fActualDt/1 -> Product3/2
  fKd/1 -> Product3/1
  Unit Delay2/1 -> Product2/1  "*fpState"
  Product2/1 -> fITerm/1, Product5/2, *fpState/1  "*fpState"
  Sum4/1 -> Product2/2
  Constant5/1 -> Sum4/1
  Product1/1 -> Sum4/2
  fIntegratorLeakFactor/1 -> Product1/2
  Saturation Dynamic/1 -> Unit Delay2/1
  Add/1 -> Saturation Dynamic/2  "fpState"
  Switch2/1 -> Product/1  "fErrorForIntegrator"
  Constant4/1 -> Switch2/1
  OR3/1 -> Switch2/2
  OR2/1 -> OR3/2
  OR1/1 -> OR3/1
  GreaterThan6/1 -> OR2/2
  GreaterThan5/1 -> OR2/1
  GreaterThan3/1 -> OR1/2
  GreaterThan4/1 -> OR1/1
  Divide1/1 -> GreaterThan4/1, Switch2/3, GreaterThan5/1  "fErrorForIntegrator"
  Constant3/1 -> GreaterThan3/2, GreaterThan4/2, GreaterThan5/2, GreaterThan6/2
  ipInhibitTarget/1 -> GreaterThan6/1, GreaterThan3/1
  fKi/1 -> Divide1/2
  Switch1/1 -> Divide1/1  "fErrorForIntegrator"
  Constant2/1 -> Switch/1
  Constant1/1 -> Switch/3
  Constant/1 -> Switch1/3
  GreaterThan2/1 -> Switch1/2
  fBlankingMaxError/1 -> GreaterThan2/2
  Abs1/1 -> GreaterThan2/1
  GreaterThan1/1 -> Switch/2
  fLargeErrorThresholdNegative/1 -> GreaterThan1/2
  fLargeErrorThresholdPositive/1 -> GreaterThan/2
  Divide/1 -> Abs1/1, Switch1/1, GreaterThan1/1, GreaterThan/1, Product4/2  "fError"
  Sign/1 -> Divide/2
  Saturation/1 -> Divide/1
  Sum2/1 -> Saturation/1  "fTemp"
  fErrorReduction/1 -> Sum2/1
  Abs/1 -> Sum2/2
  fActual/1 -> Sum22/1
  fOutMax/1 -> Saturation Dynamic1/1
  fpState/1 -> Add/2
  Saturation Dynamic1/1 -> fOutput/1
  fTarget/1 -> Sum22/2
  Product/1 -> Add/1
  Sum22/1 -> Abs/1, Sign/1  "fError"
  fOutMin/1 -> Saturation Dynamic1/3
  fIntMax/1 -> Saturation Dynamic/1
  fLoopDt/1 -> Product/2, Product1/1
  fIntMin/1 -> Saturation Dynamic/3

== system Target_Control_System/Target_Control_System/MainLoop/tiltMotor_mainLoop/Decimation gate for 200 Hz Tilt/motorTaskMainDecimationAStep(&oTilt)/Forced current injection for broken input sensors/Enabled Subsystem/Pure_0rpm_holding_mode ==
  Enable : EnablePort
  Constant : Constant  Value=0  OutDataTypeStr=single  SampleTime=-1
  Data Store Write4 : DataStoreWrite  DataStoreName=oTilt  DataStoreElements=oTilt.oMot_.oState_.oRampDataOmegaERef_.fSetpoint_  IndexOptions=Index vector (dialog)  Indices=1  OutputSizes=1
  Data Store Write5 : DataStoreWrite  DataStoreName=oTilt  DataStoreElements=oTilt.oMot_.oState_.oRampDataOmegaERef_.fRampOut_  IndexOptions=Index vector (dialog)  Indices=1  OutputSizes=1
  wires:
  Constant/1 -> Data Store Write4/1, Data Store Write5/1
